simulink library "f14actuator"  (Simulink 7.6)
settings: Solver=ode45  SolverMode=SingleTasking  StartTime=0.0  StopTime=10.0  RelTol=1e-3
values from neighbouring files (symbols this model uses):
  Ta = 0.05    [f14_digital_data.mat]    (also in f14dat_digital.m)
libraries: f14actuator x1
Description:
  | Configurable subsystem for linear and nonlinear actuators for the f14_digital model
settings Model: Creator=The MathWorks Inc.  ExtModeAutoUpdateStatusClock=off

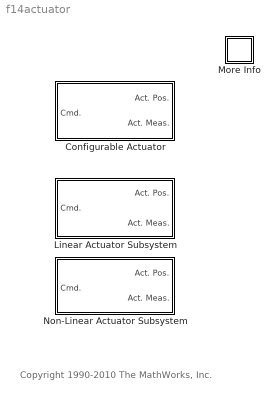
== system f14actuator ==
  note: Copyright 1990-2010 The MathWorks, Inc.
  Configurable Actuator : Subsystem  BlockChoice=Linear Actuator Subsystem
      settings: TemplateBlock=self  MemberBlocks=Linear Actuator Subsystem,Non-Linear Actuator Subsystem
  Linear Actuator Subsystem : Subsystem
      mask Display: text(0.5,0.5,'[Linear]','horizontalAlignment','center');
  More Info : Subsystem
      settings: OpenFcn=showdemo('sldemo_f14dig_script')
      mask Display: disp('?')
  Non-Linear Actuator Subsystem : Subsystem
      mask Display: text(0.5,0.5,'[Non-Linear]','horizontalAlignment','center')

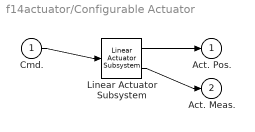
== system f14actuator/Configurable Actuator ==
  Cmd. : Inport
  Linear Actuator Subsystem : f14actuator/Linear Actuator Subsystem
  Act. Pos. : Outport
  Act. Meas. : Outport  Port=2
  wires:
  Cmd./1 -> Linear Actuator Subsystem/1
  Linear Actuator Subsystem/1 -> Act. Pos./1
  Linear Actuator Subsystem/2 -> Act. Meas./1

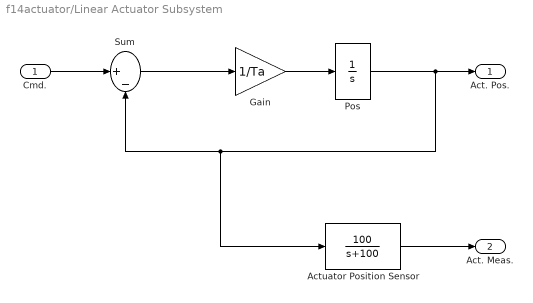
== system f14actuator/Linear Actuator Subsystem ==
  Cmd. : Inport
  Actuator Position Sensor : TransferFcn  Numerator=[100]  Denominator=[1 100]
  Gain : Gain  Gain=1/Ta  SaturateOnIntegerOverflow=on  OutDataTypeStr=Inherit: Same as input  ParamDataTypeStr=Inherit: Same as input
  Pos : Integrator  UpperSaturationLimit=pi*45/180  LowerSaturationLimit=-pi*45/180
  Sum : Sum  Inputs=|+-  SaturateOnIntegerOverflow=on  InputSameDT=on  OutDataTypeStr=Inherit: Same as first input
  Act. Pos. : Outport  InitialOutput=0
  Act. Meas. : Outport  Port=2  InitialOutput=0
  wires:
  Actuator Position Sensor/1 -> Act. Meas./1
  Cmd./1 -> Sum/1
  Pos/1 -> Act. Pos./1, Actuator Position Sensor/1, Sum/2
  Gain/1 -> Pos/1
  Sum/1 -> Gain/1

== system f14actuator/More Info ==

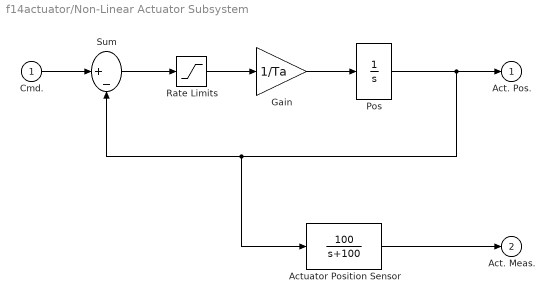
== system f14actuator/Non-Linear Actuator Subsystem ==
  Cmd. : Inport
  Actuator Position Sensor : TransferFcn  Numerator=[100]  Denominator=[1 100]
  Gain : Gain  Gain=1/Ta  SaturateOnIntegerOverflow=on  OutDataTypeStr=Inherit: Same as input  ParamDataTypeStr=Inherit: Same as input
  Pos : Integrator  LimitOutput=on  UpperSaturationLimit=pi*45/180  LowerSaturationLimit=-pi*45/180
  Rate Limits : Saturate
  Sum : Sum  Inputs=|+-  SaturateOnIntegerOverflow=on  InputSameDT=on  OutDataTypeStr=Inherit: Same as first input
  Act. Pos. : Outport  InitialOutput=0
  Act. Meas. : Outport  Port=2  InitialOutput=0
  wires:
  Actuator Position Sensor/1 -> Act. Meas./1
  Pos/1 -> Act. Pos./1, Actuator Position Sensor/1, Sum/2
  Cmd./1 -> Sum/1
  Sum/1 -> Rate Limits/1
  Gain/1 -> Pos/1
  Rate Limits/1 -> Gain/1
